simulink model "case1"  (R2024b)
settings: Solver=FixedStepAuto  StartTime=0  StopTime=1  FixedStep=1e-7  RelTol=1e-3
values from neighbouring files (symbols this model uses):
  SG_D_1_D = 0.01056    [IEEE9_case_parameters.m]    (also in case1_parameters.m; case2_parameters.m; case3_parameters.m; case4_parameters.m)
  SG_D_1_EnableSaturation = 0    [IEEE9_case_parameters.m]    (also in case1_parameters.m; case2_parameters.m; case3_parameters.m; case4_parameters.m)
  SG_D_1_f0 = 60    [IEEE9_case_parameters.m]    (also in case1_parameters.m; case2_parameters.m; case3_parameters.m; case4_parameters.m)
  SG_D_1_H = 7.5    [IEEE9_case_parameters.m]    (also in case1_parameters.m; case2_parameters.m; case3_parameters.m; case4_parameters.m)
  SG_D_1_K_A = 20    [IEEE9_case_parameters.m]    (also in case1_parameters.m; case2_parameters.m; case3_parameters.m; case4_parameters.m)
  SG_D_1_K_E = 1.000000e+1    (= 10)    [IEEE9_case_parameters.m]    (also in case1_parameters.m; case2_parameters.m; case3_parameters.m; case4_parameters.m)
  SG_D_1_K_F = 2.363    [IEEE9_case_parameters.m]    (also in case1_parameters.m; case2_parameters.m; case3_parameters.m; case4_parameters.m)
  SG_D_1_K_s = 0.5    [IEEE9_case_parameters.m]    (also in case1_parameters.m = 5; case2_parameters.m = 5; case3_parameters.m = 5; case4_parameters.m = 5)
  SG_D_1_R_a = 0.001088    [IEEE9_case_parameters.m]    (also in case1_parameters.m; case2_parameters.m; case3_parameters.m; case4_parameters.m)
  SG_D_1_S_A = 1    [IEEE9_case_parameters.m]    (also in case1_parameters.m; case2_parameters.m; case3_parameters.m; case4_parameters.m)
  SG_D_1_S_B = 0.103    [IEEE9_case_parameters.m]    (also in case1_parameters.m; case2_parameters.m; case3_parameters.m; case4_parameters.m)
  SG_D_1_S_N = 10.659857    [IEEE9_case_parameters.m]    (also in case1_parameters.m; case2_parameters.m; case3_parameters.m; case4_parameters.m)
  SG_D_1_SpeedPara = 200    [IEEE9_case_parameters.m]    (also in case1_parameters.m; case2_parameters.m; case3_parameters.m; case4_parameters.m)
  SG_D_1_T_0 = 0.720173    [IEEE9_case_parameters.m]    (also in case1_parameters.m = 0.755522; case2_parameters.m = 0.808931; case3_parameters.m = 0.869402; case4_parameters.m = 0.729316)
  SG_D_1_T_1 = 0.3    [IEEE9_case_parameters.m]    (also in case1_parameters.m; case2_parameters.m; case3_parameters.m; case4_parameters.m)
  SG_D_1_T_2 = 0.05    [IEEE9_case_parameters.m]    (also in case1_parameters.m; case2_parameters.m; case3_parameters.m; case4_parameters.m)
  SG_D_1_T_3 = 0.02    [IEEE9_case_parameters.m]    (also in case1_parameters.m; case2_parameters.m; case3_parameters.m; case4_parameters.m)
  SG_D_1_T_4 = 0.005    [IEEE9_case_parameters.m]    (also in case1_parameters.m; case2_parameters.m; case3_parameters.m; case4_parameters.m)
  SG_D_1_T_A = 0.02    [IEEE9_case_parameters.m]    (also in case1_parameters.m; case2_parameters.m; case3_parameters.m; case4_parameters.m)
  SG_D_1_T_dd = 8.000000e+0    (= 8)    [IEEE9_case_parameters.m]    (also in case1_parameters.m; case2_parameters.m; case3_parameters.m; case4_parameters.m)
  SG_D_1_T_ddd = 0.04    [IEEE9_case_parameters.m]    (also in case1_parameters.m; case2_parameters.m; case3_parameters.m; case4_parameters.m)
  SG_D_1_T_E = 0.314    [IEEE9_case_parameters.m]    (also in case1_parameters.m; case2_parameters.m; case3_parameters.m; case4_parameters.m)
  SG_D_1_T_F = 0.35    [IEEE9_case_parameters.m]    (also in case1_parameters.m; case2_parameters.m; case3_parameters.m; case4_parameters.m)
  SG_D_1_T_qd = 0.8    [IEEE9_case_parameters.m]    (also in case1_parameters.m; case2_parameters.m; case3_parameters.m; case4_parameters.m)
  SG_D_1_T_qdd = 0.02    [IEEE9_case_parameters.m]    (also in case1_parameters.m; case2_parameters.m; case3_parameters.m; case4_parameters.m)
  SG_D_1_T_speed = 0.1    [IEEE9_case_parameters.m]    (also in case1_parameters.m = 200; case2_parameters.m = 200; case3_parameters.m = 200; case4_parameters.m = 200)
  SG_D_1_T_w = 0.5    [IEEE9_case_parameters.m]    (also in case1_parameters.m; case2_parameters.m; case3_parameters.m; case4_parameters.m)
  SG_D_1_V_ref = 1.990276    [IEEE9_case_parameters.m]    (also in case1_parameters.m = 2.042296; case2_parameters.m = 2.051388; case3_parameters.m = 2.089584; case4_parameters.m = 2.01845)
  SG_D_1_w_ref = 376.991118    [IEEE9_case_parameters.m]    (also in case1_parameters.m; case2_parameters.m; case3_parameters.m; case4_parameters.m)
  SG_D_1_wb = 6.000000e+1    (= 60)    [IEEE9_case_parameters.m]    (also in case1_parameters.m; case2_parameters.m; case3_parameters.m; case4_parameters.m)
  SG_D_1_x_d = 1.9    [IEEE9_case_parameters.m]    (also in case1_parameters.m; case2_parameters.m; case3_parameters.m; case4_parameters.m)
  SG_D_1_x_dd = 0.302    [IEEE9_case_parameters.m]    (also in case1_parameters.m; case2_parameters.m; case3_parameters.m; case4_parameters.m)
  SG_D_1_x_ddd = 0.204    [IEEE9_case_parameters.m]    (also in case1_parameters.m; case2_parameters.m; case3_parameters.m; case4_parameters.m)
  SG_D_1_x_l = 0.05    [IEEE9_case_parameters.m]    (also in case1_parameters.m; case2_parameters.m; case3_parameters.m; case4_parameters.m)
  SG_D_1_x_q = 1.3    [IEEE9_case_parameters.m]    (also in case1_parameters.m; case2_parameters.m; case3_parameters.m; case4_parameters.m)
  SG_D_1_x_qd = 0.5    [IEEE9_case_parameters.m]    (also in case1_parameters.m; case2_parameters.m; case3_parameters.m; case4_parameters.m)
  SG_D_1_x_qdd = 0.3    [IEEE9_case_parameters.m]    (also in case1_parameters.m; case2_parameters.m; case3_parameters.m; case4_parameters.m)
  SG_D_2_D = 0.02    [IEEE9_case_parameters.m]    (also in case1_parameters.m; case2_parameters.m; case3_parameters.m; case4_parameters.m)
  SG_D_2_EnableSaturation = 0    [IEEE9_case_parameters.m]    (also in case1_parameters.m; case2_parameters.m; case3_parameters.m; case4_parameters.m)
  SG_D_2_f0 = 60    [IEEE9_case_parameters.m]    (also in case1_parameters.m; case2_parameters.m; case3_parameters.m; case4_parameters.m)
  SG_D_2_H = 8.000000e+0    (= 8)    [IEEE9_case_parameters.m]    (also in case1_parameters.m; case2_parameters.m; case3_parameters.m; case4_parameters.m)
  SG_D_2_K_A = 20    [IEEE9_case_parameters.m]    (also in case1_parameters.m; case2_parameters.m; case3_parameters.m; case4_parameters.m)
  SG_D_2_K_E = 1.000000e+1    (= 10)    [IEEE9_case_parameters.m]    (also in case1_parameters.m; case2_parameters.m; case3_parameters.m; case4_parameters.m)
  SG_D_2_K_F = 2.363    [IEEE9_case_parameters.m]    (also in case1_parameters.m; case2_parameters.m; case3_parameters.m; case4_parameters.m)
  SG_D_2_K_s = 0.5    [IEEE9_case_parameters.m]    (also in case1_parameters.m = 4; case2_parameters.m = 4; case3_parameters.m = 4; case4_parameters.m = 4)
  SG_D_2_R_a = 0.001088    [IEEE9_case_parameters.m]    (also in case1_parameters.m; case2_parameters.m; case3_parameters.m; case4_parameters.m)
  SG_D_2_S_A = 1    [IEEE9_case_parameters.m]    (also in case1_parameters.m; case2_parameters.m; case3_parameters.m; case4_parameters.m)
  SG_D_2_S_B = 0.103    [IEEE9_case_parameters.m]    (also in case1_parameters.m; case2_parameters.m; case3_parameters.m; case4_parameters.m)
  SG_D_2_S_N = 10.659857    [IEEE9_case_parameters.m]    (also in case1_parameters.m; case2_parameters.m; case3_parameters.m; case4_parameters.m)
  SG_D_2_SpeedPara = 200    [IEEE9_case_parameters.m]    (also in case1_parameters.m; case2_parameters.m; case3_parameters.m; case4_parameters.m)
  SG_D_2_T_0 = 1.632913    [IEEE9_case_parameters.m]    (also in case1_parameters.m = 1.632925; case2_parameters.m = 1.632915; case3_parameters.m = 1.632914; case4_parameters.m = 1.632927)
  SG_D_2_T_1 = 0.2    [IEEE9_case_parameters.m]    (also in case1_parameters.m; case2_parameters.m; case3_parameters.m; case4_parameters.m)
  SG_D_2_T_2 = 0.05    [IEEE9_case_parameters.m]    (also in case1_parameters.m; case2_parameters.m; case3_parameters.m; case4_parameters.m)
  SG_D_2_T_3 = 0.02    [IEEE9_case_parameters.m]    (also in case1_parameters.m; case2_parameters.m; case3_parameters.m; case4_parameters.m)
  SG_D_2_T_4 = 0.005    [IEEE9_case_parameters.m]    (also in case1_parameters.m; case2_parameters.m; case3_parameters.m; case4_parameters.m)
  SG_D_2_T_A = 0.02    [IEEE9_case_parameters.m]    (also in case1_parameters.m; case2_parameters.m; case3_parameters.m; case4_parameters.m)
  SG_D_2_T_dd = 7.9    [IEEE9_case_parameters.m]    (also in case1_parameters.m; case2_parameters.m; case3_parameters.m; case4_parameters.m)
  SG_D_2_T_ddd = 0.04    [IEEE9_case_parameters.m]    (also in case1_parameters.m; case2_parameters.m; case3_parameters.m; case4_parameters.m)
  SG_D_2_T_E = 0.314    [IEEE9_case_parameters.m]    (also in case1_parameters.m; case2_parameters.m; case3_parameters.m; case4_parameters.m)
  SG_D_2_T_F = 0.35    [IEEE9_case_parameters.m]    (also in case1_parameters.m; case2_parameters.m; case3_parameters.m; case4_parameters.m)
  SG_D_2_T_qd = 0.8    [IEEE9_case_parameters.m]    (also in case1_parameters.m; case2_parameters.m; case3_parameters.m; case4_parameters.m)
  SG_D_2_T_qdd = 0.015    [IEEE9_case_parameters.m]    (also in case1_parameters.m; case2_parameters.m; case3_parameters.m; case4_parameters.m)
  SG_D_2_T_speed = 0.1    [IEEE9_case_parameters.m]    (also in case1_parameters.m = 150; case2_parameters.m = 150; case3_parameters.m = 150; case4_parameters.m = 150)
  SG_D_2_T_w = 0.35    [IEEE9_case_parameters.m]    (also in case1_parameters.m; case2_parameters.m; case3_parameters.m; case4_parameters.m)
  SG_D_2_V_ref = 2.58547    [IEEE9_case_parameters.m]    (also in case1_parameters.m = 2.597896; case2_parameters.m = 2.587136; case3_parameters.m = 2.586042; case4_parameters.m = 2.599679)
  SG_D_2_w_ref = 376.991118    [IEEE9_case_parameters.m]    (also in case1_parameters.m; case2_parameters.m; case3_parameters.m; case4_parameters.m)
  SG_D_2_wb = 6.000000e+1    (= 60)    [IEEE9_case_parameters.m]    (also in case1_parameters.m; case2_parameters.m; case3_parameters.m; case4_parameters.m)
  SG_D_2_x_d = 1.8    [IEEE9_case_parameters.m]    (also in case1_parameters.m; case2_parameters.m; case3_parameters.m; case4_parameters.m)
  SG_D_2_x_dd = 0.302    [IEEE9_case_parameters.m]    (also in case1_parameters.m; case2_parameters.m; case3_parameters.m; case4_parameters.m)
  SG_D_2_x_ddd = 0.204    [IEEE9_case_parameters.m]    (also in case1_parameters.m; case2_parameters.m; case3_parameters.m; case4_parameters.m)
  SG_D_2_x_l = 0.05    [IEEE9_case_parameters.m]    (also in case1_parameters.m; case2_parameters.m; case3_parameters.m; case4_parameters.m)
  SG_D_2_x_q = 1.25    [IEEE9_case_parameters.m]    (also in case1_parameters.m; case2_parameters.m; case3_parameters.m; case4_parameters.m)
  SG_D_2_x_qd = 0.5    [IEEE9_case_parameters.m]    (also in case1_parameters.m; case2_parameters.m; case3_parameters.m; case4_parameters.m)
  SG_D_2_x_qdd = 0.3    [IEEE9_case_parameters.m]    (also in case1_parameters.m; case2_parameters.m; case3_parameters.m; case4_parameters.m)
  SG_D_3_D = 0.02    [IEEE9_case_parameters.m]    (also in case1_parameters.m; case2_parameters.m; case3_parameters.m; case4_parameters.m)
  SG_D_3_EnableSaturation = 0    [IEEE9_case_parameters.m]    (also in case1_parameters.m; case2_parameters.m; case3_parameters.m; case4_parameters.m)
  SG_D_3_f0 = 60    [IEEE9_case_parameters.m]    (also in case1_parameters.m; case2_parameters.m; case3_parameters.m; case4_parameters.m)
  SG_D_3_H = 7.7    [IEEE9_case_parameters.m]    (also in case1_parameters.m; case2_parameters.m; case3_parameters.m; case4_parameters.m)
  SG_D_3_K_A = 20    [IEEE9_case_parameters.m]    (also in case1_parameters.m; case2_parameters.m; case3_parameters.m; case4_parameters.m)
  SG_D_3_K_E = 1.000000e+1    (= 10)    [IEEE9_case_parameters.m]    (also in case1_parameters.m; case2_parameters.m; case3_parameters.m; case4_parameters.m)
  SG_D_3_K_F = 2.363    [IEEE9_case_parameters.m]    (also in case1_parameters.m; case2_parameters.m; case3_parameters.m; case4_parameters.m)
  SG_D_3_K_s = 0.2    [IEEE9_case_parameters.m]    (also in case1_parameters.m = 2; case2_parameters.m = 2; case3_parameters.m = 2; case4_parameters.m = 2)
  SG_D_3_R_a = 0.001088    [IEEE9_case_parameters.m]    (also in case1_parameters.m; case2_parameters.m; case3_parameters.m; case4_parameters.m)
  SG_D_3_S_A = 1    [IEEE9_case_parameters.m]    (also in case1_parameters.m; case2_parameters.m; case3_parameters.m; case4_parameters.m)
  SG_D_3_S_B = 0.103    [IEEE9_case_parameters.m]    (also in case1_parameters.m; case2_parameters.m; case3_parameters.m; case4_parameters.m)
  SG_D_3_S_N = 10.659857    [IEEE9_case_parameters.m]    (also in case1_parameters.m; case2_parameters.m; case3_parameters.m; case4_parameters.m)
  SG_D_3_SpeedPara = 200    [IEEE9_case_parameters.m]    (also in case1_parameters.m; case2_parameters.m; case3_parameters.m; case4_parameters.m)
  SG_D_3_T_0 = 0.850788    [IEEE9_case_parameters.m]    (also in case1_parameters.m = 0.850786; case2_parameters.m = 0.850787; case3_parameters.m; case4_parameters.m = 0.850786)
  SG_D_3_T_1 = 0.2    [IEEE9_case_parameters.m]    (also in case1_parameters.m; case2_parameters.m; case3_parameters.m; case4_parameters.m)
  SG_D_3_T_2 = 0.05    [IEEE9_case_parameters.m]    (also in case1_parameters.m; case2_parameters.m; case3_parameters.m; case4_parameters.m)
  SG_D_3_T_3 = 0.02    [IEEE9_case_parameters.m]    (also in case1_parameters.m; case2_parameters.m; case3_parameters.m; case4_parameters.m)
  SG_D_3_T_4 = 0.005    [IEEE9_case_parameters.m]    (also in case1_parameters.m; case2_parameters.m; case3_parameters.m; case4_parameters.m)
  SG_D_3_T_A = 0.02    [IEEE9_case_parameters.m]    (also in case1_parameters.m; case2_parameters.m; case3_parameters.m; case4_parameters.m)
  SG_D_3_T_dd = 8.1    [IEEE9_case_parameters.m]    (also in case1_parameters.m; case2_parameters.m; case3_parameters.m; case4_parameters.m)
  SG_D_3_T_ddd = 0.04    [IEEE9_case_parameters.m]    (also in case1_parameters.m; case2_parameters.m; case3_parameters.m; case4_parameters.m)
  SG_D_3_T_E = 0.314    [IEEE9_case_parameters.m]    (also in case1_parameters.m; case2_parameters.m; case3_parameters.m; case4_parameters.m)
  SG_D_3_T_F = 0.35    [IEEE9_case_parameters.m]    (also in case1_parameters.m; case2_parameters.m; case3_parameters.m; case4_parameters.m)
  SG_D_3_T_qd = 0.8    [IEEE9_case_parameters.m]    (also in case1_parameters.m; case2_parameters.m; case3_parameters.m; case4_parameters.m)
  SG_D_3_T_qdd = 0.015    [IEEE9_case_parameters.m]    (also in case1_parameters.m; case2_parameters.m; case3_parameters.m; case4_parameters.m)
  SG_D_3_T_speed = 0.1    [IEEE9_case_parameters.m]    (also in case1_parameters.m = 180; case2_parameters.m = 180; case3_parameters.m = 180; case4_parameters.m = 180)
  SG_D_3_T_w = 0.4    [IEEE9_case_parameters.m]    (also in case1_parameters.m; case2_parameters.m; case3_parameters.m; case4_parameters.m)
  SG_D_3_V_ref = 1.892727    [IEEE9_case_parameters.m]    (also in case1_parameters.m = 1.906439; case2_parameters.m = 1.895535; case3_parameters.m = 1.892105; case4_parameters.m = 1.906598)
  SG_D_3_w_ref = 376.991118    [IEEE9_case_parameters.m]    (also in case1_parameters.m; case2_parameters.m; case3_parameters.m; case4_parameters.m)
  SG_D_3_wb = 6.000000e+1    (= 60)    [IEEE9_case_parameters.m]    (also in case1_parameters.m; case2_parameters.m; case3_parameters.m; case4_parameters.m)
  SG_D_3_x_d = 1.85    [IEEE9_case_parameters.m]    (also in case1_parameters.m; case2_parameters.m; case3_parameters.m; case4_parameters.m)
  SG_D_3_x_dd = 0.302    [IEEE9_case_parameters.m]    (also in case1_parameters.m; case2_parameters.m; case3_parameters.m; case4_parameters.m)
  SG_D_3_x_ddd = 0.204    [IEEE9_case_parameters.m]    (also in case1_parameters.m; case2_parameters.m; case3_parameters.m; case4_parameters.m)
  SG_D_3_x_l = 0.05    [IEEE9_case_parameters.m]    (also in case1_parameters.m; case2_parameters.m; case3_parameters.m; case4_parameters.m)
  SG_D_3_x_q = 1.2    [IEEE9_case_parameters.m]    (also in case1_parameters.m; case2_parameters.m; case3_parameters.m; case4_parameters.m)
  SG_D_3_x_qd = 0.5    [IEEE9_case_parameters.m]    (also in case1_parameters.m; case2_parameters.m; case3_parameters.m; case4_parameters.m)
  SG_D_3_x_qdd = 0.3    [IEEE9_case_parameters.m]    (also in case1_parameters.m; case2_parameters.m; case3_parameters.m; case4_parameters.m)
(part 6 of 12)

== system case1/SG_D_1/d_psi_kq_SG_D_1_block ==
  note: d_psi_kq_SG_D_1 in case1
      | $-\frac{\psi _{\mathrm{gq},\mathrm{SG},D,1}+\psi _{\mathrm{kq},\mathrm{SG},D,1}+\frac{\left(x_{l}-x_{\mathrm{qd}}\right)\,\left(\psi _{q,\mathrm{SG},D,1}+\frac{\psi _{\mathrm{gq},\mathrm{SG},D,1}\,\left(x_{l}-x_{\mathrm{qdd}}\right)}{x_{l}-x_{\mathrm{qd}}}+\frac{\psi _{\mathrm{kq},\mathrm{SG},D,1}\,\left(x_{\mathrm{qd}}-x_{\mathrm{qdd}}\right)}{x_{l}-x_{\mathrm{qd}}}\right)}{x_{\mathrm{qdd}}}}{T_{\mathrm{qdd}}}$
      | Automatically generated on 2025-10-31 18:47:16 .
  State_psi_gq_SG_D_1_5db4b : Inport
  State_psi_kq_SG_D_1_f7f57 : Inport  Port=2
  State_psi_gq_SG_D_1_83c8c : Inport  Port=3
  State_psi_kq_SG_D_1_b0ad3 : Inport  Port=4
  State_psi_q_SG_D_1_db3ff : Inport  Port=5
  Add_116b7 : Sum
  Add_2e38b : Sum
  Add_2ef19 : Sum
  Add_648d6 : Sum
  Add_73bbb : Sum
  Add_83a04 : Sum
  Constant_-1_273d7 : Constant  Value=-1
  Constant_-1_a16ed : Constant  Value=-1
  Constant_-1_ae179 : Constant  Value=-1
  Constant_-1_c5c44 : Constant  Value=-1
  Constant_-1_ed5a6 : Constant  Value=-1
  Constant_T_qdd_7098b : Constant  Value=T_qdd
  Constant_x_l_1d8b2 : Constant  Value=x_l
  Constant_x_l_34694 : Constant  Value=x_l
  Constant_x_l_7c861 : Constant  Value=x_l
  Constant_x_l_d0a3c : Constant  Value=x_l
  Constant_x_qd_54c19 : Constant  Value=x_qd
  Constant_x_qd_809b7 : Constant  Value=x_qd
  Constant_x_qd_a4dda : Constant  Value=x_qd
  Constant_x_qd_bfbcb : Constant  Value=x_qd
  Constant_x_qdd_241fa : Constant  Value=x_qdd
  Constant_x_qdd_5d64a : Constant  Value=x_qdd
  Constant_x_qdd_ca32a : Constant  Value=x_qdd
  Divide_0ee25 : Product  Inputs=*/
  Divide_44dc9 : Product  Inputs=*/
  Divide_6685c : Product  Inputs=*/
  Divide_ae4e7 : Product  Inputs=*/
  Product_09a80 : Product
  Product_1c9ba : Product
  Product_928a2 : Product
  Product_b0c46 : Product
  Product_b455e : Product
  Product_b975e : Product
  Product_e3999 : Product
  Product_e7277 : Product
  Subtract_60067 : Sum  Inputs=+-
  Subtract_890b3 : Sum  Inputs=+-
  Subtract_a524f : Sum  Inputs=+-
  Blockout_d_psi_kq_SG_D_1_8a28d : Outport
  wires:
  Product_e3999/1 -> Add_116b7/1
  Constant_-1_a16ed/1 -> Product_e3999/1
  Constant_x_l_1d8b2/1 -> Product_e3999/2
  Constant_x_qdd_ca32a/1 -> Add_116b7/2
  Constant_-1_273d7/1 -> Product_b975e/1
  Constant_x_qd_a4dda/1 -> Subtract_a524f/1
  Constant_x_qd_54c19/1 -> Add_648d6/2
  Constant_-1_c5c44/1 -> Product_b0c46/1
  Constant_x_l_7c861/1 -> Product_b975e/2
  Constant_x_qdd_5d64a/1 -> Subtract_a524f/2
  Constant_x_qd_bfbcb/1 -> Add_2ef19/2
  Constant_x_l_d0a3c/1 -> Product_b0c46/2
  Subtract_890b3/1 -> Add_83a04/1
  Product_1c9ba/1 -> Subtract_890b3/1
  State_psi_gq_SG_D_1_83c8c/1 -> Product_09a80/1
  Add_116b7/1 -> Product_09a80/2
  Product_b0c46/1 -> Add_2e38b/1
  Constant_x_qd_809b7/1 -> Add_2e38b/2
  State_psi_kq_SG_D_1_b0ad3/1 -> Product_928a2/1
  Product_b975e/1 -> Add_2ef19/1
  Subtract_a524f/1 -> Product_928a2/2
  Product_09a80/1 -> Divide_6685c/1
  Add_2e38b/1 -> Divide_6685c/2
  Product_928a2/1 -> Divide_ae4e7/1
  Add_2ef19/1 -> Divide_ae4e7/2
  Constant_-1_ae179/1 -> Product_e7277/1
  Constant_x_l_34694/1 -> Product_e7277/2
  Divide_6685c/1 -> Subtract_60067/1
  Divide_ae4e7/1 -> Subtract_60067/2
  Product_e7277/1 -> Add_648d6/1
  Add_73bbb/1 -> Product_b455e/2
  Subtract_60067/1 -> Add_73bbb/1
  State_psi_q_SG_D_1_db3ff/1 -> Add_73bbb/2
  Constant_-1_ed5a6/1 -> Product_1c9ba/1
  State_psi_gq_SG_D_1_5db4b/1 -> Product_1c9ba/2
  Divide_0ee25/1 -> Add_83a04/2
  Product_b455e/1 -> Divide_0ee25/1
  Add_648d6/1 -> Product_b455e/1
  State_psi_kq_SG_D_1_f7f57/1 -> Subtract_890b3/2
  Constant_x_qdd_241fa/1 -> Divide_0ee25/2
  Add_83a04/1 -> Divide_44dc9/1
  Constant_T_qdd_7098b/1 -> Divide_44dc9/2
  Divide_44dc9/1 -> Blockout_d_psi_kq_SG_D_1_8a28d/1

== system case1/SG_D_1/d_psi_q_SG_D_1_block ==
  note: d_psi_q_SG_D_1 in case1
      | $2\,\pi \,f_{0}\,\left(v_{d,\mathrm{SG},D,1}\,\cos\left(\theta _{\mathrm{SG},D,1}\right)+v_{q,\mathrm{SG},D,1}\,\sin\left(\theta _{\mathrm{SG},D,1}\right)-\frac{R_{a}\,\left(\psi _{q,\mathrm{SG},D,1}+\frac{\psi _{\mathrm{gq},\mathrm{SG},D,1}\,\left(x_{l}-x_{\mathrm{qdd}}\right)}{x_{l}-x_{\mathrm{qd}}}+\frac{\psi _{\mathrm{kq},\mathrm{SG},D,1}\,\left(x_{\mathrm{qd}}-x_{\mathrm{qdd}}\right)}{x_{l}-x_{\mathrm{qd}}}\right)}{x_{\mathrm{qdd}}}-\frac{\psi _{d,\mathrm{SG},D,1}\,w_{\mathrm{SG},D,1}}{2\,f_{0}\,\pi }\right)$
      | Automatically generated on 2025-10-31 18:47:02 .
  State_psi_gq_SG_D_1_c29fe : Inport
  State_psi_kq_SG_D_1_bac7c : Inport  Port=2
  State_psi_q_SG_D_1_1d0c2 : Inport  Port=3
  Input_v_d_SG_D_1_f7fec : Inport  Port=4
  State_theta_SG_D_1_d73f5 : Inport  Port=5
  Input_v_q_SG_D_1_145b1 : Inport  Port=6
  State_theta_SG_D_1_fb557 : Inport  Port=7
  State_psi_d_SG_D_1_00025 : Inport  Port=8
  State_w_SG_D_1_8f4a2 : Inport  Port=9
  Add_4d064 : Sum
  Add_68451 : Sum
  Add_7c2a3 : Sum
  Add_8bb9d : Sum
  Add_c3baf : Sum
  Constant_-1_13315 : Constant  Value=-1
  Constant_-1_dfd9e : Constant  Value=-1
  Constant_-1_e6efe : Constant  Value=-1
  Constant_-2.0_dbd21 : Constant  Value=-2.0
  Constant_2.0_4a36d : Constant  Value=2.0
  Constant_R_a_1e160 : Constant  Value=R_a
  Constant_f0_684d5 : Constant  Value=f0
  Constant_f0_97970 : Constant  Value=f0
  Constant_pi_49e5e : Constant  Value=pi
  Constant_pi_9ab14 : Constant  Value=pi
  Constant_x_l_325fe : Constant  Value=x_l
  Constant_x_l_7c6b2 : Constant  Value=x_l
  Constant_x_l_d0cb9 : Constant  Value=x_l
  Constant_x_qd_62520 : Constant  Value=x_qd
  Constant_x_qd_b9dc9 : Constant  Value=x_qd
  Constant_x_qd_d0a38 : Constant  Value=x_qd
  Constant_x_qdd_147cd : Constant  Value=x_qdd
  Constant_x_qdd_f1c73 : Constant  Value=x_qdd
  Constant_x_qdd_f6b40 : Constant  Value=x_qdd
  Divide_12493 : Product  Inputs=*/
  Divide_23e4a : Product  Inputs=*/
  Divide_51eae : Product  Inputs=*/
  Divide_5d20e : Product  Inputs=*/
  MathFunc_cos_c3f9b : Trigonometry  Operator=cos
  MathFunc_sin_1725b : Trigonometry
  Product_021c0 : Product
  Product_5581f : Product
  Product_56851 : Product
  Product_5863e : Product
  Product_5bab2 : Product
  Product_67689 : Product
  Product_86a8d : Product
  Product_9d02a : Product
  Product_ace16 : Product
  Product_b7a78 : Product
  Product_c8c51 : Product
  Product_cf47c : Product
  Product_e2306 : Product
  Product_f68ff : Product
  Subtract_1987b : Sum  Inputs=+-
  Subtract_46e63 : Sum  Inputs=+-
  Subtract_9d106 : Sum  Inputs=+-
  Subtract_fd00d : Sum  Inputs=+-
  Blockout_d_psi_q_SG_D_1_1eeca : Outport
  wires:
  Divide_51eae/1 -> Subtract_fd00d/1
  Product_5863e/1 -> Add_4d064/1
  Constant_x_l_7c6b2/1 -> Product_5863e/2
  Constant_-1_dfd9e/1 -> Product_5863e/1
  Constant_x_qdd_147cd/1 -> Add_4d064/2
  Constant_x_l_325fe/1 -> Product_9d02a/2
  Constant_-1_13315/1 -> Product_9d02a/1
  Constant_x_l_d0cb9/1 -> Product_86a8d/2
  Constant_x_qdd_f6b40/1 -> Subtract_1987b/2
  State_psi_kq_SG_D_1_bac7c/1 -> Product_ace16/1
  Constant_-1_e6efe/1 -> Product_86a8d/1
  Constant_x_qd_b9dc9/1 -> Subtract_1987b/1
  State_psi_gq_SG_D_1_c29fe/1 -> Product_56851/1
  Product_5581f/1 -> Blockout_d_psi_q_SG_D_1_1eeca/1
  Subtract_fd00d/1 -> Add_68451/1
  Product_56851/1 -> Divide_51eae/1
  Add_4d064/1 -> Product_56851/2
  Divide_12493/1 -> Subtract_fd00d/2
  Product_9d02a/1 -> Add_8bb9d/1
  Constant_x_qd_62520/1 -> Add_8bb9d/2
  Constant_-2.0_dbd21/1 -> Product_e2306/1
  Product_ace16/1 -> Divide_12493/1
  Product_86a8d/1 -> Add_c3baf/1
  Subtract_1987b/1 -> Product_ace16/2
  Constant_x_qd_d0a38/1 -> Add_c3baf/2
  Add_8bb9d/1 -> Divide_51eae/2
  Add_c3baf/1 -> Divide_12493/2
  Constant_f0_97970/1 -> Product_67689/2
  State_psi_q_SG_D_1_1d0c2/1 -> Add_68451/2
  Product_cf47c/1 -> Product_021c0/1
  Constant_R_a_1e160/1 -> Product_b7a78/1
  Product_021c0/1 -> Divide_23e4a/2
  Product_b7a78/1 -> Divide_5d20e/1
  Add_68451/1 -> Product_b7a78/2
  State_theta_SG_D_1_d73f5/1 -> MathFunc_cos_c3f9b/1
  Input_v_d_SG_D_1_f7fec/1 -> Product_5bab2/1
  Constant_x_qdd_f1c73/1 -> Divide_5d20e/2
  MathFunc_cos_c3f9b/1 -> Product_5bab2/2
  State_theta_SG_D_1_fb557/1 -> MathFunc_sin_1725b/1
  Divide_5d20e/1 -> Subtract_9d106/1
  Constant_2.0_4a36d/1 -> Product_cf47c/1
  State_w_SG_D_1_8f4a2/1 -> Product_c8c51/2
  Constant_pi_49e5e/1 -> Product_cf47c/2
  Subtract_46e63/1 -> Add_7c2a3/1
  Product_5bab2/1 -> Subtract_9d106/2
  Divide_23e4a/1 -> Add_7c2a3/2
  Input_v_q_SG_D_1_145b1/1 -> Product_f68ff/1
  MathFunc_sin_1725b/1 -> Product_f68ff/2
  Product_f68ff/1 -> Subtract_46e63/2
  State_psi_d_SG_D_1_00025/1 -> Product_c8c51/1
  Constant_f0_684d5/1 -> Product_021c0/2
  Constant_pi_9ab14/1 -> Product_e2306/2
  Subtract_9d106/1 -> Subtract_46e63/1
  Product_c8c51/1 -> Divide_23e4a/1
  Product_e2306/1 -> Product_67689/1
  Product_67689/1 -> Product_5581f/1
  Add_7c2a3/1 -> Product_5581f/2

== system case1/SG_D_1/d_theta_SG_D_1_block ==
  note: d_theta_SG_D_1 in case1
      | $w_{\mathrm{SG},D,1}-2\,\pi \,f_{0}$
      | Automatically generated on 2025-10-31 18:47:23 .
  State_w_SG_D_1_1349a : Inport
  Add_68325 : Sum
  Constant_-2.0_165a7 : Constant  Value=-2.0
  Constant_f0_1c2a1 : Constant  Value=f0
  Constant_pi_59ceb : Constant  Value=pi
  Product_44a6b : Product
  Product_92915 : Product
  Blockout_d_theta_SG_D_1_0d12b : Outport
  wires:
  State_w_SG_D_1_1349a/1 -> Add_68325/2
  Constant_-2.0_165a7/1 -> Product_44a6b/1
  Constant_f0_1c2a1/1 -> Product_92915/2
  Constant_pi_59ceb/1 -> Product_44a6b/2
  Product_92915/1 -> Add_68325/1
  Product_44a6b/1 -> Product_92915/1
  Add_68325/1 -> Blockout_d_theta_SG_D_1_0d12b/1

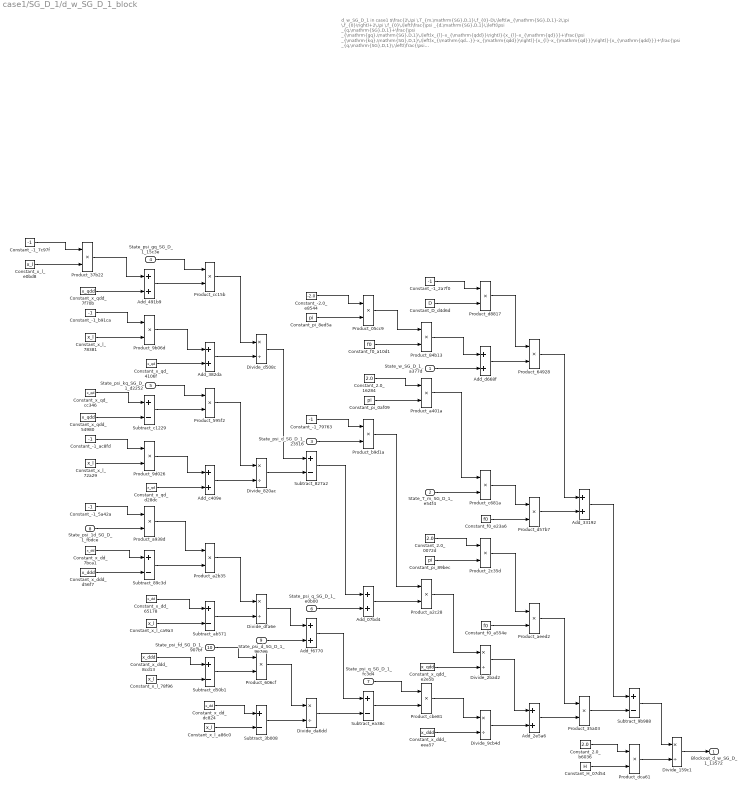
== system case1/SG_D_1/d_w_SG_D_1_block ==
  note: d_w_SG_D_1 in case1
      | $\frac{2\,\pi \,T_{m,\mathrm{SG},D,1}\,f_{0}-D\,\left(w_{\mathrm{SG},D,1}-2\,\pi \,f_{0}\right)+2\,\pi \,f_{0}\,\left(\frac{\psi _{d,\mathrm{SG},D,1}\,\left(\psi _{q,\mathrm{SG},D,1}+\frac{\psi _{\mathrm{gq},\mathrm{SG},D,1}\,\left(x_{l}-x_{\mathrm{qdd}}\right)}{x_{l}-x_{\mathrm{qd}}}+\frac{\psi _{\mathrm{kq},\mathrm{SG},D,1}\,\left(x_{\mathrm{qd}}-x_{\mathrm{qdd}}\right)}{x_{l}-x_{\mathrm{qd}}}\right)}{x_{\mathrm{qdd}}}+\frac{\psi _{q,\mathrm{SG},D,1}\,\left(\frac{\psi _{\mathrm{1d},\mathrm{SG},D,1}\,\left(x_{\mathrm{dd}}-x_{\mathrm{ddd}}\right)}{x_{\mathrm{dd}}-x_{l}}-\psi _{d,\mathrm{SG},D,1}+\frac{\psi _{\mathrm{fd},\mathrm{SG},D,1}\,\left(x_{\mathrm{ddd}}-x_{l}\right)}{x_{\mathrm{dd}}-x_{l}}\right)}{x_{\mathrm{ddd}}}\right)}{2\,H}$
      | Automatically generated on 2025-10-31 18:47:22 .
  State_w_SG_D_1_a377d : Inport
  State_T_m_SG_D_1_e54f4 : Inport  Port=2
  State_psi_d_SG_D_1_23516 : Inport  Port=3
  State_psi_gq_SG_D_1_15c3e : Inport  Port=4
  State_psi_kq_SG_D_1_d2252 : Inport  Port=5
  State_psi_q_SG_D_1_e0b00 : Inport  Port=6
  State_psi_q_SG_D_1_fc3d4 : Inport  Port=7
  State_psi_1d_SG_D_1_fbdce : Inport  Port=8
  State_psi_d_SG_D_1_9e7e6 : Inport  Port=9
  State_psi_fd_SG_D_1_907bf : Inport  Port=10
  Add_07bd4 : Sum
  Add_2e5a6 : Sum
  Add_33192 : Sum
  Add_382da : Sum
  Add_491b9 : Sum
  Add_c409e : Sum
  Add_d668f : Sum
  Add_f6770 : Sum
  Constant_-1_2a7f0 : Constant  Value=-1
  Constant_-1_5a42a : Constant  Value=-1
  Constant_-1_79763 : Constant  Value=-1
  Constant_-1_7c97f : Constant  Value=-1
  Constant_-1_ac8fd : Constant  Value=-1
  Constant_-1_b91ca : Constant  Value=-1
  Constant_-2.0_e8544 : Constant  Value=-2.0
  Constant_2.0_0072d : Constant  Value=2.0
  Constant_2.0_16284 : Constant  Value=2.0
  Constant_2.0_b6036 : Constant  Value=2.0
  Constant_D_d4d6d : Constant  Value=D
  Constant_H_07d54 : Constant  Value=H
  Constant_f0_a10d1 : Constant  Value=f0
  Constant_f0_a554e : Constant  Value=f0
  Constant_f0_e23a6 : Constant  Value=f0
  Constant_pi_0af09 : Constant  Value=pi
  Constant_pi_89bec : Constant  Value=pi
  Constant_pi_8ed5a : Constant  Value=pi
  Constant_x_dd_65178 : Constant  Value=x_dd
  Constant_x_dd_7bca1 : Constant  Value=x_dd
  Constant_x_dd_dc824 : Constant  Value=x_dd
  Constant_x_ddd_8cd13 : Constant  Value=x_ddd
  Constant_x_ddd_d56f7 : Constant  Value=x_ddd
  Constant_x_ddd_eea57 : Constant  Value=x_ddd
  Constant_x_l_72a29 : Constant  Value=x_l
  Constant_x_l_78381 : Constant  Value=x_l
  Constant_x_l_78f96 : Constant  Value=x_l
  Constant_x_l_a86c0 : Constant  Value=x_l
  Constant_x_l_ca9a3 : Constant  Value=x_l
  Constant_x_l_e0bd8 : Constant  Value=x_l
  Constant_x_qd_4106f : Constant  Value=x_qd
  Constant_x_qd_cc346 : Constant  Value=x_qd
  Constant_x_qd_d28dc : Constant  Value=x_qd
  Constant_x_qdd_54980 : Constant  Value=x_qdd
  Constant_x_qdd_7f70b : Constant  Value=x_qdd
  Constant_x_qdd_e2e5b : Constant  Value=x_qdd
  Divide_159c1 : Product  Inputs=*/
  Divide_2bad2 : Product  Inputs=*/
  Divide_820ac : Product  Inputs=*/
  Divide_9cb4d : Product  Inputs=*/
  Divide_d508c : Product  Inputs=*/
  Divide_da6dd : Product  Inputs=*/
  Divide_dfa6e : Product  Inputs=*/
  Product_05cc9 : Product
  Product_2c35d : Product
  Product_35a03 : Product
  Product_37b22 : Product
  Product_595f2 : Product
  Product_606cf : Product
  Product_64928 : Product
  Product_84b13 : Product
  Product_9b06d : Product
  Product_9d026 : Product
  Product_a2b35 : Product
  Product_a2c28 : Product
  Product_a401a : Product
  Product_a938d : Product
  Product_aeed2 : Product
  Product_b9d1a : Product
  Product_c681a : Product
  Product_cbe81 : Product
  Product_cc15b : Product
  Product_d57b7 : Product
  Product_d8817 : Product
  Product_dca61 : Product
  Subtract_3b008 : Sum  Inputs=+-
  Subtract_827a2 : Sum  Inputs=+-
  Subtract_89c3d : Sum  Inputs=+-
  Subtract_9b988 : Sum  Inputs=+-
  Subtract_ab571 : Sum  Inputs=+-
  Subtract_c1229 : Sum  Inputs=+-
  Subtract_d50b1 : Sum  Inputs=+-
  Subtract_ea38c : Sum  Inputs=+-
  Blockout_d_w_SG_D_1_13572 : Outport
  wires:
  Product_84b13/1 -> Add_d668f/1
  Constant_-1_7c97f/1 -> Product_37b22/1
  Constant_pi_0af09/1 -> Product_a401a/2
  Constant_x_qdd_7f70b/1 -> Add_491b9/2
  Constant_x_l_e0bd8/1 -> Product_37b22/2
  Product_37b22/1 -> Add_491b9/1
  Constant_x_qd_cc346/1 -> Subtract_c1229/1
  Constant_-1_b91ca/1 -> Product_9b06d/1
  Product_05cc9/1 -> Product_84b13/1
  Constant_x_qdd_54980/1 -> Subtract_c1229/2
  State_psi_q_SG_D_1_fc3d4/1 -> Product_cbe81/1
  Constant_x_l_78381/1 -> Product_9b06d/2
  Constant_-1_ac8fd/1 -> Product_9d026/1
  Constant_x_l_72a29/1 -> Product_9d026/2
  Constant_-1_5a42a/1 -> Product_a938d/1
  Product_9b06d/1 -> Add_382da/1
  State_psi_1d_SG_D_1_fbdce/1 -> Product_a938d/2
  Constant_x_dd_7bca1/1 -> Subtract_89c3d/1
  Subtract_c1229/1 -> Product_595f2/2
  Constant_x_ddd_d56f7/1 -> Subtract_89c3d/2
  State_psi_gq_SG_D_1_15c3e/1 -> Product_cc15b/1
  Product_b9d1a/1 -> Product_a2c28/1
  Add_491b9/1 -> Product_cc15b/2
  Constant_x_qd_4106f/1 -> Add_382da/2
  State_psi_kq_SG_D_1_d2252/1 -> Product_595f2/1
  Constant_f0_a10d1/1 -> Product_84b13/2
  Product_9d026/1 -> Add_c409e/1
  Constant_x_dd_65178/1 -> Subtract_ab571/1
  Constant_x_qd_d28dc/1 -> Add_c409e/2
  Product_a938d/1 -> Product_a2b35/1
  Subtract_89c3d/1 -> Product_a2b35/2
  Constant_x_l_ca9a3/1 -> Subtract_ab571/2
  Constant_x_ddd_8cd13/1 -> Subtract_d50b1/1
  Constant_x_l_78f96/1 -> Subtract_d50b1/2
  State_w_SG_D_1_a377d/1 -> Add_d668f/2
  Divide_2bad2/1 -> Add_2e5a6/1
  Constant_-1_2a7f0/1 -> Product_d8817/1
  Product_cc15b/1 -> Divide_d508c/1
  Add_d668f/1 -> Product_64928/2
  Divide_d508c/1 -> Subtract_827a2/1
  Add_382da/1 -> Divide_d508c/2
  Constant_pi_8ed5a/1 -> Product_05cc9/2
  Product_595f2/1 -> Divide_820ac/1
  Add_c409e/1 -> Divide_820ac/2
  Product_a2b35/1 -> Divide_dfa6e/1
  Divide_dfa6e/1 -> Add_f6770/1
  Subtract_ab571/1 -> Divide_dfa6e/2
  State_psi_fd_SG_D_1_907bf/1 -> Product_606cf/1
  Subtract_d50b1/1 -> Product_606cf/2
  Constant_x_dd_dc824/1 -> Subtract_3b008/1
  Constant_x_l_a86c0/1 -> Subtract_3b008/2
  Divide_820ac/1 -> Subtract_827a2/2
  Constant_2.0_16284/1 -> Product_a401a/1
  State_psi_d_SG_D_1_9e7e6/1 -> Add_f6770/2
  Product_606cf/1 -> Divide_da6dd/1
  Subtract_3b008/1 -> Divide_da6dd/2
  Constant_-2.0_e8544/1 -> Product_05cc9/1
  Constant_-1_79763/1 -> Product_b9d1a/1
  State_psi_d_SG_D_1_23516/1 -> Product_b9d1a/2
  Subtract_827a2/1 -> Add_07bd4/1
  Subtract_ea38c/1 -> Product_cbe81/2
  State_psi_q_SG_D_1_e0b00/1 -> Add_07bd4/2
  Add_f6770/1 -> Subtract_ea38c/1
  Divide_da6dd/1 -> Subtract_ea38c/2
  Add_07bd4/1 -> Product_a2c28/2
  Constant_D_d4d6d/1 -> Product_d8817/2
  Product_a401a/1 -> Product_c681a/1
  State_T_m_SG_D_1_e54f4/1 -> Product_c681a/2
  Constant_2.0_0072d/1 -> Product_2c35d/1
  Constant_pi_89bec/1 -> Product_2c35d/2
  Product_a2c28/1 -> Divide_2bad2/1
  Constant_x_qdd_e2e5b/1 -> Divide_2bad2/2
  Product_cbe81/1 -> Divide_9cb4d/1
  Constant_x_ddd_eea57/1 -> Divide_9cb4d/2
  Product_d8817/1 -> Product_64928/1
  Product_c681a/1 -> Product_d57b7/1
  Constant_f0_e23a6/1 -> Product_d57b7/2
  Product_2c35d/1 -> Product_aeed2/1
  Constant_f0_a554e/1 -> Product_aeed2/2
  Divide_9cb4d/1 -> Add_2e5a6/2
  Product_64928/1 -> Add_33192/1
  Product_d57b7/1 -> Add_33192/2
  Product_aeed2/1 -> Product_35a03/1
  Add_2e5a6/1 -> Product_35a03/2
  Add_33192/1 -> Subtract_9b988/1
  Product_35a03/1 -> Subtract_9b988/2
  Constant_2.0_b6036/1 -> Product_dca61/1
  Constant_H_07d54/1 -> Product_dca61/2
  Subtract_9b988/1 -> Divide_159c1/1
  Product_dca61/1 -> Divide_159c1/2
  Divide_159c1/1 -> Blockout_d_w_SG_D_1_13572/1

== system case1/SG_D_1/i_d_SG_D_1_block ==
  note: i_d_SG_D_1 in case1
      | $\frac{\sin\left(\theta _{\mathrm{SG},D,1}\right)\,\left(\frac{\psi _{\mathrm{1d},\mathrm{SG},D,1}\,\left(x_{\mathrm{dd}}-x_{\mathrm{ddd}}\right)}{x_{\mathrm{dd}}-x_{l}}-\psi _{d,\mathrm{SG},D,1}+\frac{\psi _{\mathrm{fd},\mathrm{SG},D,1}\,\left(x_{\mathrm{ddd}}-x_{l}\right)}{x_{\mathrm{dd}}-x_{l}}\right)}{x_{\mathrm{ddd}}}-\frac{\cos\left(\theta _{\mathrm{SG},D,1}\right)\,\left(\psi _{q,\mathrm{SG},D,1}+\frac{\psi _{\mathrm{gq},\mathrm{SG},D,1}\,\left(x_{l}-x_{\mathrm{qdd}}\right)}{x_{l}-x_{\mathrm{qd}}}+\frac{\psi _{\mathrm{kq},\mathrm{SG},D,1}\,\left(x_{\mathrm{qd}}-x_{\mathrm{qdd}}\right)}{x_{l}-x_{\mathrm{qd}}}\right)}{x_{\mathrm{qdd}}}$
      | Automatically generated on 2025-10-31 18:47:46 .
  State_psi_gq_SG_D_1_4d36f : Inport
  State_psi_kq_SG_D_1_5abe0 : Inport  Port=2
  State_psi_q_SG_D_1_b5d7f : Inport  Port=3
  State_theta_SG_D_1_47360 : Inport  Port=4
  State_psi_1d_SG_D_1_a973f : Inport  Port=5
  State_psi_d_SG_D_1_2da12 : Inport  Port=6
  State_psi_fd_SG_D_1_52673 : Inport  Port=7
  State_theta_SG_D_1_0c5f1 : Inport  Port=8
  Add_30a6b : Sum
  Add_3460c : Sum
  Add_a9246 : Sum
  Add_b9f4b : Sum
  Add_e5b49 : Sum
  Constant_-1_40724 : Constant  Value=-1
  Constant_-1_6867a : Constant  Value=-1
  Constant_-1_82f9b : Constant  Value=-1
  Constant_-1_9f2f2 : Constant  Value=-1
  Constant_-1_c5244 : Constant  Value=-1
  Constant_x_dd_1399a : Constant  Value=x_dd
  Constant_x_dd_28243 : Constant  Value=x_dd
  Constant_x_dd_8492e : Constant  Value=x_dd
  Constant_x_ddd_2bb5a : Constant  Value=x_ddd
  Constant_x_ddd_7d405 : Constant  Value=x_ddd
  Constant_x_ddd_85714 : Constant  Value=x_ddd
  Constant_x_l_26bbe : Constant  Value=x_l
  Constant_x_l_35483 : Constant  Value=x_l
  Constant_x_l_38784 : Constant  Value=x_l
  Constant_x_l_9d1d7 : Constant  Value=x_l
  Constant_x_l_c351b : Constant  Value=x_l
  Constant_x_l_c8087 : Constant  Value=x_l
  Constant_x_qd_2c4b7 : Constant  Value=x_qd
  Constant_x_qd_38467 : Constant  Value=x_qd
  Constant_x_qd_b62ac : Constant  Value=x_qd
  Constant_x_qdd_093e5 : Constant  Value=x_qdd
  Constant_x_qdd_88c83 : Constant  Value=x_qdd
  Constant_x_qdd_cf8f7 : Constant  Value=x_qdd
  Divide_040af : Product  Inputs=*/
  Divide_1592c : Product  Inputs=*/
  Divide_45e1b : Product  Inputs=*/
  Divide_94b90 : Product  Inputs=*/
  Divide_d9696 : Product  Inputs=*/
  Divide_ea568 : Product  Inputs=*/
  MathFunc_cos_66ba2 : Trigonometry  Operator=cos
  MathFunc_sin_8dceb : Trigonometry
  Product_0196e : Product
  Product_22140 : Product
  Product_43740 : Product
  Product_5ea4f : Product
  Product_5eab4 : Product
  Product_8dd19 : Product
  Product_98f71 : Product
  Product_a3dbf : Product
  Product_b0052 : Product
  Product_ce6d7 : Product
  Product_f4981 : Product
  Subtract_03554 : Sum  Inputs=+-
  Subtract_15c4d : Sum  Inputs=+-
  Subtract_210b8 : Sum  Inputs=+-
  Subtract_3b634 : Sum  Inputs=+-
  Subtract_46972 : Sum  Inputs=+-
  Subtract_a9d4b : Sum  Inputs=+-
  Subtract_f5f5e : Sum  Inputs=+-
  Subtract_fdb13 : Sum  Inputs=+-
  Blockout_i_d_SG_D_1_13e50 : Outport
  wires:
  Constant_-1_82f9b/1 -> Product_5eab4/1
  Constant_x_l_c351b/1 -> Product_5eab4/2
  Constant_x_ddd_2bb5a/1 -> Subtract_15c4d/2
  Product_5eab4/1 -> Add_a9246/1
  Constant_x_qdd_cf8f7/1 -> Subtract_fdb13/2
  Constant_x_l_38784/1 -> Product_98f71/2
  Constant_x_qd_38467/1 -> Add_b9f4b/2
  Constant_x_qdd_093e5/1 -> Add_a9246/2
  Constant_x_qd_b62ac/1 -> Subtract_fdb13/1
  MathFunc_cos_66ba2/1 -> Product_5ea4f/2
  Constant_-1_40724/1 -> Product_98f71/1
  Constant_-1_c5244/1 -> Product_43740/1
  Subtract_46972/1 -> Blockout_i_d_SG_D_1_13e50/1
  Constant_x_l_26bbe/1 -> Product_43740/2
  Divide_d9696/1 -> Subtract_f5f5e/1
  State_psi_gq_SG_D_1_4d36f/1 -> Product_22140/1
  Subtract_03554/1 -> Product_0196e/2
  Add_a9246/1 -> Product_22140/2
  Divide_1592c/1 -> Add_30a6b/1
  Product_98f71/1 -> Add_3460c/1
  Constant_x_qd_2c4b7/1 -> Add_3460c/2
  State_psi_kq_SG_D_1_5abe0/1 -> Product_ce6d7/1
  Add_30a6b/1 -> Subtract_210b8/1
  Add_3460c/1 -> Divide_d9696/2
  Subtract_fdb13/1 -> Product_ce6d7/2
  Product_43740/1 -> Add_b9f4b/1
  Constant_-1_6867a/1 -> Product_f4981/1
  State_psi_1d_SG_D_1_a973f/1 -> Product_f4981/2
  Constant_x_dd_28243/1 -> Subtract_15c4d/1
  Product_22140/1 -> Divide_d9696/1
  Product_8dd19/1 -> Divide_94b90/1
  Subtract_15c4d/1 -> Product_a3dbf/2
  Product_ce6d7/1 -> Divide_45e1b/1
  Product_f4981/1 -> Product_a3dbf/1
  Add_b9f4b/1 -> Divide_45e1b/2
  Constant_x_dd_1399a/1 -> Subtract_a9d4b/1
  Subtract_f5f5e/1 -> Add_e5b49/1
  Constant_x_l_35483/1 -> Subtract_a9d4b/2
  Constant_x_ddd_7d405/1 -> Subtract_03554/1
  Constant_x_l_c8087/1 -> Subtract_03554/2
  Divide_94b90/1 -> Subtract_46972/2
  Divide_45e1b/1 -> Subtract_f5f5e/2
  State_theta_SG_D_1_47360/1 -> MathFunc_cos_66ba2/1
  Product_a3dbf/1 -> Divide_1592c/1
  Subtract_a9d4b/1 -> Divide_1592c/2
  State_theta_SG_D_1_0c5f1/1 -> MathFunc_sin_8dceb/1
  State_psi_fd_SG_D_1_52673/1 -> Product_0196e/1
  Constant_x_dd_8492e/1 -> Subtract_3b634/1
  Constant_x_l_9d1d7/1 -> Subtract_3b634/2
  State_psi_q_SG_D_1_b5d7f/1 -> Add_e5b49/2
  State_psi_d_SG_D_1_2da12/1 -> Add_30a6b/2
  Constant_x_ddd_85714/1 -> Divide_94b90/2
  MathFunc_sin_8dceb/1 -> Product_8dd19/2
  Product_0196e/1 -> Divide_ea568/1
  Constant_-1_9f2f2/1 -> Product_b0052/1
  Subtract_3b634/1 -> Divide_ea568/2
  Add_e5b49/1 -> Product_b0052/2
  Divide_ea568/1 -> Subtract_210b8/2
  Product_b0052/1 -> Product_5ea4f/1
  Subtract_210b8/1 -> Product_8dd19/1
  Constant_x_qdd_88c83/1 -> Divide_040af/2
  Product_5ea4f/1 -> Divide_040af/1
  Divide_040af/1 -> Subtract_46972/1

== system case1/SG_D_1/i_q_SG_D_1_block ==
  note: i_q_SG_D_1 in case1
      | $-\frac{\sin\left(\theta _{\mathrm{SG},D,1}\right)\,\left(\psi _{q,\mathrm{SG},D,1}+\frac{\psi _{\mathrm{gq},\mathrm{SG},D,1}\,\left(x_{l}-x_{\mathrm{qdd}}\right)}{x_{l}-x_{\mathrm{qd}}}+\frac{\psi _{\mathrm{kq},\mathrm{SG},D,1}\,\left(x_{\mathrm{qd}}-x_{\mathrm{qdd}}\right)}{x_{l}-x_{\mathrm{qd}}}\right)}{x_{\mathrm{qdd}}}-\frac{\cos\left(\theta _{\mathrm{SG},D,1}\right)\,\left(\frac{\psi _{\mathrm{1d},\mathrm{SG},D,1}\,\left(x_{\mathrm{dd}}-x_{\mathrm{ddd}}\right)}{x_{\mathrm{dd}}-x_{l}}-\psi _{d,\mathrm{SG},D,1}+\frac{\psi _{\mathrm{fd},\mathrm{SG},D,1}\,\left(x_{\mathrm{ddd}}-x_{l}\right)}{x_{\mathrm{dd}}-x_{l}}\right)}{x_{\mathrm{ddd}}}$
      | Automatically generated on 2025-10-31 18:47:51 .
  State_psi_gq_SG_D_1_ff441 : Inport
  State_psi_kq_SG_D_1_4e43a : Inport  Port=2
  State_psi_q_SG_D_1_65128 : Inport  Port=3
  State_theta_SG_D_1_2a693 : Inport  Port=4
  State_psi_1d_SG_D_1_b398b : Inport  Port=5
  State_psi_d_SG_D_1_79e1a : Inport  Port=6
  State_psi_fd_SG_D_1_5070a : Inport  Port=7
  State_theta_SG_D_1_2605c : Inport  Port=8
  Add_0be34 : Sum
  Add_1bfbe : Sum
  Add_2dfa5 : Sum
  Add_870f6 : Sum
  Add_d3877 : Sum
  Add_e542d : Sum
  Constant_-1_1df96 : Constant  Value=-1
  Constant_-1_39316 : Constant  Value=-1
  Constant_-1_9e96f : Constant  Value=-1
  Constant_-1_b2aa1 : Constant  Value=-1
  Constant_-1_ec25c : Constant  Value=-1
  Constant_x_dd_15e4d : Constant  Value=x_dd
  Constant_x_dd_50932 : Constant  Value=x_dd
  Constant_x_dd_95407 : Constant  Value=x_dd
  Constant_x_ddd_5b968 : Constant  Value=x_ddd
  Constant_x_ddd_b6f12 : Constant  Value=x_ddd
  Constant_x_ddd_d1da8 : Constant  Value=x_ddd
  Constant_x_l_14408 : Constant  Value=x_l
  Constant_x_l_373c1 : Constant  Value=x_l
  Constant_x_l_4ba18 : Constant  Value=x_l
  Constant_x_l_5a324 : Constant  Value=x_l
  Constant_x_l_63c2f : Constant  Value=x_l
  Constant_x_l_7cfcd : Constant  Value=x_l
  Constant_x_qd_23192 : Constant  Value=x_qd
  Constant_x_qd_3d1d4 : Constant  Value=x_qd
  Constant_x_qd_81966 : Constant  Value=x_qd
  Constant_x_qdd_67b19 : Constant  Value=x_qdd
  Constant_x_qdd_b9c06 : Constant  Value=x_qdd
  Constant_x_qdd_f9107 : Constant  Value=x_qdd
  Divide_01975 : Product  Inputs=*/
  Divide_2e122 : Product  Inputs=*/
  Divide_7e497 : Product  Inputs=*/
  Divide_9197b : Product  Inputs=*/
  Divide_c683f : Product  Inputs=*/
  Divide_cf9e4 : Product  Inputs=*/
  MathFunc_cos_e316e : Trigonometry  Operator=cos
  MathFunc_sin_86c3e : Trigonometry
  Product_0de84 : Product
  Product_14425 : Product
  Product_3c430 : Product
  Product_42f58 : Product
  Product_7d94f : Product
  Product_97e7b : Product
  Product_9b0f6 : Product
  Product_c1717 : Product
  Product_c3613 : Product
  Product_d4ab8 : Product
  Product_f9f54 : Product
  Subtract_0240e : Sum  Inputs=+-
  Subtract_2681c : Sum  Inputs=+-
  Subtract_53604 : Sum  Inputs=+-
  Subtract_851bb : Sum  Inputs=+-
  Subtract_8bf47 : Sum  Inputs=+-
  Subtract_d37da : Sum  Inputs=+-
  Subtract_d8e74 : Sum  Inputs=+-
  Blockout_i_q_SG_D_1_39ddb : Outport
  wires:
  State_theta_SG_D_1_2605c/1 -> MathFunc_cos_e316e/1
  State_psi_fd_SG_D_1_5070a/1 -> Product_3c430/1
  Constant_-1_9e96f/1 -> Product_14425/1
  Constant_x_l_14408/1 -> Product_14425/2
  Subtract_851bb/1 -> Product_3c430/2
  Constant_x_l_373c1/1 -> Subtract_8bf47/2
  Product_14425/1 -> Add_0be34/1
  Constant_x_qdd_f9107/1 -> Add_0be34/2
  Constant_x_qd_81966/1 -> Subtract_d37da/1
  Constant_x_qdd_b9c06/1 -> Divide_01975/2
  MathFunc_sin_86c3e/1 -> Product_c3613/2
  Constant_-1_b2aa1/1 -> Product_97e7b/1
  Constant_x_qdd_67b19/1 -> Subtract_d37da/2
  Add_d3877/1 -> Product_9b0f6/2
  Product_0de84/1 -> Divide_cf9e4/1
  Constant_x_l_4ba18/1 -> Product_97e7b/2
  Constant_-1_39316/1 -> Product_f9f54/1
  Constant_x_l_5a324/1 -> Product_f9f54/2
  State_psi_gq_SG_D_1_ff441/1 -> Product_0de84/1
  Add_0be34/1 -> Product_0de84/2
  Divide_7e497/1 -> Add_2dfa5/1
  Product_97e7b/1 -> Add_870f6/1
  Divide_01975/1 -> Add_e542d/1
  Constant_x_qd_23192/1 -> Add_870f6/2
  State_psi_kq_SG_D_1_4e43a/1 -> Product_c1717/1
  Add_2dfa5/1 -> Subtract_2681c/1
  Subtract_d37da/1 -> Product_c1717/2
  Divide_cf9e4/1 -> Subtract_53604/1
  Add_870f6/1 -> Divide_cf9e4/2
  Product_f9f54/1 -> Add_1bfbe/1
  Constant_x_qd_3d1d4/1 -> Add_1bfbe/2
  Constant_-1_ec25c/1 -> Product_7d94f/1
  MathFunc_cos_e316e/1 -> Product_42f58/2
  Product_3c430/1 -> Divide_9197b/1
  State_psi_1d_SG_D_1_b398b/1 -> Product_7d94f/2
  Constant_x_l_63c2f/1 -> Subtract_0240e/2
  Constant_x_dd_95407/1 -> Subtract_d8e74/1
  Divide_9197b/1 -> Subtract_2681c/2
  Constant_x_ddd_d1da8/1 -> Subtract_d8e74/2
  Product_42f58/1 -> Divide_c683f/1
  Product_c1717/1 -> Divide_2e122/1
  Product_7d94f/1 -> Product_d4ab8/1
  Add_1bfbe/1 -> Divide_2e122/2
  Subtract_d8e74/1 -> Product_d4ab8/2
  State_psi_d_SG_D_1_79e1a/1 -> Add_2dfa5/2
  Constant_x_dd_50932/1 -> Subtract_8bf47/1
  Constant_x_ddd_5b968/1 -> Subtract_851bb/1
  Constant_x_l_7cfcd/1 -> Subtract_851bb/2
  Divide_c683f/1 -> Add_e542d/2
  Divide_2e122/1 -> Subtract_53604/2
  State_theta_SG_D_1_2a693/1 -> MathFunc_sin_86c3e/1
  Product_d4ab8/1 -> Divide_7e497/1
  Subtract_8bf47/1 -> Divide_7e497/2
  Constant_x_dd_15e4d/1 -> Subtract_0240e/1
  Subtract_53604/1 -> Add_d3877/1
  State_psi_q_SG_D_1_65128/1 -> Add_d3877/2
  Subtract_0240e/1 -> Divide_9197b/2
  Subtract_2681c/1 -> Product_42f58/1
  Constant_-1_1df96/1 -> Product_9b0f6/1
  Product_9b0f6/1 -> Product_c3613/1
  Product_c3613/1 -> Divide_01975/1
  Constant_x_ddd_b6f12/1 -> Divide_c683f/2
  Add_e542d/1 -> Blockout_i_q_SG_D_1_39ddb/1

== system case1/SG_D_1/theta_SG_D_1_out_block ==
  note: theta_SG_D_1_out in case1
      | $\theta _{\mathrm{SG},D,1}$
      | Automatically generated on 2025-10-31 18:47:57 .
  State_theta_SG_D_1_08b1b : Inport
  Blockout_theta_SG_D_1_out_85d64 : Outport
  wires:
  State_theta_SG_D_1_08b1b/1 -> Blockout_theta_SG_D_1_out_85d64/1

== system case1/SG_D_1/w_SG_D_1_out_block ==
  note: w_SG_D_1_out in case1
      | $w_{\mathrm{SG},D,1}$
      | Automatically generated on 2025-10-31 18:47:56 .
  State_w_SG_D_1_bec44 : Inport
  Blockout_w_SG_D_1_out_92872 : Outport
  wires:
  State_w_SG_D_1_bec44/1 -> Blockout_w_SG_D_1_out_92872/1
